simulink library "powerlib_modelsV2"  (Simulink 6.0)
settings: Solver=ode45  SolverMode=SingleTasking  StartTime=0.0  StopTime=10.0  RelTol=1e-3
undefined symbols (not defined in the file or in its folder): A, Ac, B, Bc, C, Cc, Cs, Current, damp, Dc, Dd, DiscIntNeverNeededParam, dref, dwo, exc, F, fb, gate, GH, GHd, GI, GId, GL, GLd, H, HT, hyd, ib, ib2, io, isfinite, j, K, Kd, Kg, L, Lad, Laq, lim, LIM, Ll, Llfd, Llkd, Llkq1, Llkq2, Llr, Lls, LowerFlux, N, N2, Nb, Nb2, nb_arm, p, Par_HarmoA_pu, Par_HarmoB_pu, Par_Timing_Harmo, Par_Timing_Variation, Par_Vps, Pb ... (+58)
libraries: powerlib_extras x14
(part 3 of 11)

== system powerlib_modelsV2/Switch Current Source ==
  IGBT : Subsystem  mask(IGBT model){Ron=0.01, Lon=1e-6, Vf=1, Tf=10e-6, Tt=20e-6, IC=0}
      mask prompts: Ron "Resistance Ron (Ohms) :"; Lon "Inductance Lon (H) :"; Vf "Forward voltage Vf (V) :"; Tf "Current 10% fall time Tf (s) :"; Tt "Current tail time Tt (s):"; IC "Initial current Ic (A) :"
      mask help: Simulink model for the IGBT blockt. In on-state, the IGBT model has an internal resistance (Ron) and an inductance (Lon). Lon cannot be set to zero. In off-state, the IGBT model has an infinite impedance. Discretization of the IGBTblock is available only through the Universal Bridge block.
  detailed_thyristor : Subsystem  mask(Thyristor model){Ron=1e-2, Lon=10e-6, Vf=0.8, IL=0.1, Tq=100e-6, IC=0}
      mask prompts: Ron "Resistance Ron (Ohms) :"; Lon "Inductance Lon (H) :"; Vf "Forward voltage Vf (V) :"; IL "Latching current Il (A) :"; Tq "Turn-off time Tq (s) :"; IC "Initial current Ic (A) :"
      mask help:
      | Simulates a thyristor in parallel with a series Rs-Cs snubber circuit. In on-state thyristor has internal resistance (Ron) and inductance (Lon - required by model, cannot be set to zero). In off-state thyristor impedance is infinite.
      |
      | Input one is Vak and input two is the gate signal .
      | Output one is Iak and output two is the measurement output vector [Iak Vak].
  diode : Subsystem  mask(Diode model){Ron=0.01, Lon=1e-6, Vf=0.8, IC=0}
      mask prompts: Ron "Resistance Ron (Ohms) :"; Lon "Inductance Lon (H) :"; Vf "Forward voltage Vf (V) :"; IC "Initial current Ic (A) :"
      mask help: Simulink model for the Diode block when Lon >0. In on-state, the diode has an internal resistance (Ron) and an inductance (Lon). Lon cannot be set to zero. In off-state, the diode impedance is infinite. Input one is Vak. Output one is Iak and output 2 is the measurement output vector [Iak Vak].
  gto : Subsystem  mask(Gto model){Ron=0.001, Lon=1e-5, Vf=0.8, Tf=200e-6, Tt=200e-6, IC=0}
      mask prompts: Ron "Resistance Ron (Ohms) :"; Lon "Inductance Lon (H) :"; Vf "Forward voltage Vf (V) :"; Tf "Current 10% fall time Tf (s) :"; Tt "Current tail time Tt (s) :"; IC "Initial current Ic (A) :"
      mask help: Simulink model for the GTO block. In on-state, the GTO has an internal resistance (Ron) and an inductance (Lon). Lon cannot be set to zero. In off-state, the GTO impedance is infinite. Input one is Vak and input two is the Gate signal. Output one is Iak and output 2 is the measurement output vector [Iak Vak].
  mosfet : Subsystem  mask(Mosfet model ){Ron=0.001, Lon=0.05, Rd=1e-6, IC=0}
      mask prompts: Ron "MOSFET resistance Ron (Ohms) :"; Lon "MOSFET inductance Lon (H) :"; Rd "Internal diode resistance Rd (Ohms) :"; IC "Initial current Ic (A) :"
      mask help: Simulink model for the MOSFETblock. the model simulate an internal diode in parallel with the MOSFET. In on-state, the MOSFET has an internal resistance (Ron if Ids>0 , Rd if Ids<0) and an inductance (Lon). Lon cannot be set to zero). In off-state, the MOSFET impedance is infinite. Input one is Vds and input two is the Gate signal. Output one is Ids and output 2 is the measurement output vector [Ids Vds].
      mask init:
      | ICmos=abs(IC).*(IC>0);
      | ICdiode=abs(IC).*(IC<0);
  thyristor : Subsystem  AncestorBlock=powerlib_models/Switch Current Source/thyristor_GS  mask(Thyristor s model){Ron=1, Lon=10e-6, Vf=0.8, IC=47e-6}
      mask prompts: Ron "Resistance Ron (Ohms) :"; Lon "Inductance Lon (H) :"; Vf "Forward voltage Vf (V) :"; IC "Initial current Ic (A) :"
      mask help: Simulink model for the Thyristor block when Lon>0. In on-state, the thyristor has an internal resistance (Ron) and an inductance (Lon). Lon cannot be set to zero. In off-state, the thyristor impedance is infinite. Input one is Vak and input two is the gate signal. Output one is Iak and output two is the measurement output vector [Iak Vak].

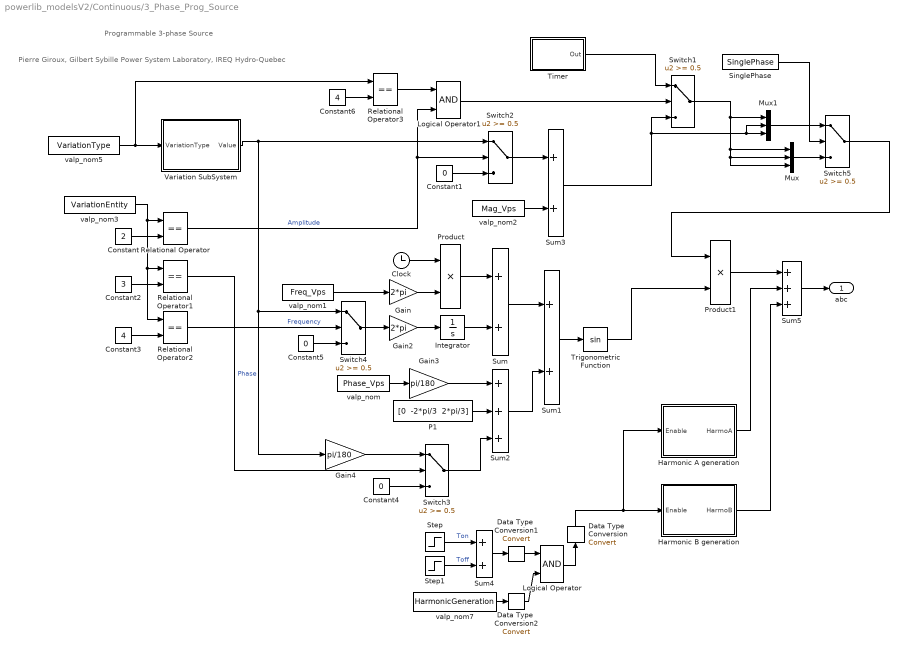
== system powerlib_modelsV2/Continuous/3_Phase_Prog_Source ==
  note: Pierre Giroux, Gilbert Sybille
      | Power System Laboratory, IREQ
      | Hydro-Quebec
  note: Programmable 3-phase Source
  Clock : Clock
  Constant : Constant  Value=2
  Constant1 : Constant  Value=0
  Constant2 : Constant  Value=3
  Constant3 : Constant  Value=4
  Constant4 : Constant  Value=0
  Constant5 : Constant  Value=0
  Constant6 : Constant  Value=4
  Data Type  Conversion : DataTypeConversion  Orientation=up  SaturateOnIntegerOverflow=on  RndMeth=Zero
  Data Type  Conversion1 : DataTypeConversion  SaturateOnIntegerOverflow=on  RndMeth=Zero
  Data Type  Conversion2 : DataTypeConversion  SaturateOnIntegerOverflow=on  RndMeth=Zero
  Gain : Gain  Gain=2*pi  SaturateOnIntegerOverflow=on
  Gain2 : Gain  Gain=2*pi  SaturateOnIntegerOverflow=on
  Gain3 : Gain  Gain=pi/180  SaturateOnIntegerOverflow=on
  Gain4 : Gain  Gain=pi/180  SaturateOnIntegerOverflow=on
  Harmonic A generation : Subsystem  mask(Harmonic generation){Freq_Vps=Freq_Vps, n_Harmo=n_HarmoA, Mag_Harmo=Mag_HarmoA, Phase_Harmo=Phase_HarmoA, Seq_Harmo=Seq_HarmoA, Ts=0}
      mask prompts: Ts "Sample time:"
  Harmonic B generation : Subsystem  mask(Harmonic generation){Freq_Vps=Freq_Vps, n_Harmo=n_HarmoB, Mag_Harmo=Mag_HarmoB, Phase_Harmo=Phase_HarmoB, Seq_Harmo=Seq_HarmoB, Ts=0}
      mask prompts: Ts "Sample time:"
  Integrator : Integrator
  Logical Operator : Logic
  Logical Operator1 : Logic
  Mux : Mux  Inputs=3
  Mux1 : Mux  Inputs=3
  P1 : Constant  Value="[0  -2*pi/3  2*pi/3]"
  Product : Product  SaturateOnIntegerOverflow=on  InputSameDT=on
  Product1 : Product  SaturateOnIntegerOverflow=on  InputSameDT=on
  Relational Operator{,1..3} (4 alike) : RelationalOperator  Operator===  InputSameDT=on
  SinglePhase : Constant  Value=SinglePhase
  Step : Step  Time=Ton_Harmo  SampleTime=0
  Step1 : Step  Time=Toff_Harmo  After=-1  SampleTime=0
  Sum{,1,3..4} (4 alike) : Sum  SaturateOnIntegerOverflow=on  InputSameDT=on
  Sum2 : Sum  Inputs=+++  SaturateOnIntegerOverflow=on  InputSameDT=on
  Sum5 : Sum  Inputs=+++  SaturateOnIntegerOverflow=on  InputSameDT=on
  Switch{1..5} (5 alike) : Switch  Threshold=0.5  InputSameDT=on
  Timer : Subsystem  mask(Timer){t=Xtime, e=Yampli, Ts=0}
      mask prompts: t "Time (s):"; e "Amplitude:"; Ts "Sample time (s)"
      mask help:
      | Generates a signal changing  at specified times.
      |
      | Value of the signal at time zero must  be specified.
      mask init:
      | tt=t;sv=e;
      | tv=[-1,tt(1),reshape(repmat(reshape(tt(2:end),1,length(tt)-1),2,1),1,2*length(tt)-2),tt(end)+1];
      | %sv=(sv(:)'~=0);
      | opv=[sv(1),reshape(repmat(sv(1:end-1),2,1),1,2*length(sv)-2),sv(end),sv(end)];
      mask Display: plot( tv(2:end-1), opv(2:end-1) )
  Trigonometric Function : Trigonometry
  Variation SubSystem : Subsystem  mask(Variation Subsystem){VariationStep=VariationStep, VariationRate=VariationRate, VariationFreq=VariationFreq, VariationMag=VariationMag, Ton_Variation=Ton_Variation, Toff_Variation=Toff_Variation, Ts=0}
      mask prompts: Ts "Sample time:"
  valp_nom : Constant  Value=Phase_Vps
  valp_nom1 : Constant  Value=Freq_Vps
  valp_nom2 : Constant  Value=Mag_Vps
  valp_nom3 : Constant  Value=VariationEntity
  valp_nom5 : Constant  Value=VariationType
  valp_nom7 : Constant  Value=HarmonicGeneration
  abc : Outport  InitialOutput=0
  wires:
  Logical Operator1/1 -> Switch1/2
  Relational Operator3/1 -> Logical Operator1/1
  Switch5/1 -> Product1/1
  Switch1/1 -> Mux1/1, Mux/3, Mux/2, Mux/1
  Mux/1 -> Switch5/3
  SinglePhase/1 -> Switch5/2
  Mux1/1 -> Switch5/1
  Timer/1(Out) -> Switch1/1
  Sum3/1 -> Mux1/2, Mux1/3, Switch1/3
  Constant6/1 -> Relational Operator3/2
  Gain4/1 -> Switch3/1
  Harmonic B generation/1(HarmoB) -> Sum5/3
  Step1/1 -> Sum4/2  "Toff"
  Step/1 -> Sum4/1  "Ton"
  Sum5/1 -> abc/1
  Harmonic A generation/1(HarmoA) -> Sum5/2
  Constant5/1 -> Switch4/3
  Constant3/1 -> Relational Operator2/2
  Constant2/1 -> Relational Operator1/2
  valp_nom3/1 -> Relational Operator1/1, Relational Operator2/1, Relational Operator/1
  Constant/1 -> Relational Operator/2
  Relational Operator2/1 -> Switch4/2  "Frequency"
  Switch4/1 -> Gain2/1
  Variation SubSystem/1(Value) -> Gain4/1, Switch4/1, Switch2/1
  Relational Operator1/1 -> Switch3/2  "Phase"
  Constant4/1 -> Switch3/3
  Switch3/1 -> Sum2/3
  valp_nom5/1 -> Relational Operator3/1, Variation SubSystem/1(VariationType)
  Relational Operator/1 -> Logical Operator1/2, Switch2/2  "Amplitude"
  valp_nom2/1 -> Sum3/2
  Sum2/1 -> Sum1/2
  Constant1/1 -> Switch2/3
  Switch2/1 -> Sum3/1
  Product1/1 -> Sum5/1
  valp_nom1/1 -> Gain/1
  valp_nom/1 -> Gain3/1
  Gain3/1 -> Sum2/1
  Trigonometric Function/1 -> Product1/2
  P1/1 -> Sum2/2
  Integrator/1 -> Sum/2
  Gain2/1 -> Integrator/1
  Sum1/1 -> Trigonometric Function/1
  Sum/1 -> Sum1/1
  Clock/1 -> Product/1
  Gain/1 -> Product/2
  Product/1 -> Sum/1
  Logical Operator/1 -> Data Type  Conversion/1
  Data Type  Conversion/1 -> Harmonic A generation/1(Enable), Harmonic B generation/1(Enable)
  Sum4/1 -> Data Type  Conversion1/1
  Data Type  Conversion1/1 -> Logical Operator/1
  valp_nom7/1 -> Data Type  Conversion2/1
  Data Type  Conversion2/1 -> Logical Operator/2

== system powerlib_modelsV2/Continuous/3_phase_source ==
  Constant : Constant  Value=complex(A*cos(P*pi/180),A*sin(P*pi/180))
  Constant1 : Constant  Value=complex(A*cos((P-120)*pi/180),A*sin((P-120)*pi/180))
  Constant2 : Constant  Value=complex(A*cos((P+120)*pi/180),A*sin((P+120)*pi/180))
  Mux : Mux  Inputs=6
  Sine Wave : Sin  Amplitude=A  Frequency=2*pi*F  Phase=P*pi/180  SampleTime=0
  Sine Wave1 : Sin  Amplitude=A  Frequency=2*pi*F  Phase=(P-120)*pi/180  SampleTime=0
  Sine Wave2 : Sin  Amplitude=A  Frequency=2*pi*F  Phase=(P+120)*pi/180  SampleTime=0
  Out1 : Outport
  wires:
  Constant/1 -> Mux/2
  Sine Wave/1 -> Mux/1
  Sine Wave1/1 -> Mux/3
  Constant1/1 -> Mux/4
  Sine Wave2/1 -> Mux/5
  Constant2/1 -> Mux/6
  Mux/1 -> Out1/1

== system powerlib_modelsV2/Continuous/Dynamic_Load ==
  v : Inport  Port=1  LatchInput=off
  PQ : Inport  Port=2  LatchInput=off
  3-phase PLL1 : Subsystem  mask(3-phase PLL){Par_Init=[Pha_V0  fnom], ParK=[60 1400]}
      mask prompts: Par_Init "Initial inputs:[ Phase(degrees)   Frequency(Hz) ]"; ParK "Regulator gains [ Kp  Ki ]"
      mask help:
      | This Phase Locked Loop (PLL) system can be used  to synchronize on a set of variable frequency, three-phase sinusoidal signals.
      |
      | Input 1: Vector containing the normalized
      |              three-phase signals [Va Vb Vc]
      | Output 1:  Measured frequency (Hz) = w/(2pi)
      | Output 2:  Ramp w.t   varying between  0 and 2*pi,
      | synchronized on zero crossings of the fundamental (positive-sequence) of phase A.
      | Output 3: Vector [sin(wt) cos(wt)]
      mask init:
      | Kp=ParK(1);
      | Ki=ParK(2);
      | Phase_Init=Par_Init(1);
      | Finit=Par_Init(2);
  Break  Alg. Loop : Subsystem  Orientation=left
  Complex to Real-Imag : ComplexToRealImag  Orientation=left
  Demux : Demux  Outputs=2
  Ground : Ground  Orientation=left
  Mux1 : Mux  Orientation=left  Inputs=3
  Positive Sequence  current : Subsystem
  Real-Imag to Complex : RealImagToComplex
  Real-Imag to Complex1 : RealImagToComplex
  Selector : Selector  Orientation=left  Elements=1:2  InputPortWidth=3
  V> pu : Gain  Gain=1/Vbase  SaturateOnIntegerOverflow=on
  Variable Frequency Mean value1 : Subsystem  mask(Variable-Frequency Mean Value){Finit=fnom, Vinit=Mag_V0}
      mask prompts: Finit "Initial frequency (Hz):"; Vinit "Initial input (DC component):"
      mask help:
      | This  block computes the mean value of the input signal (port In) over a running window of one cycle of a specified frequency (port Freq).
      |
      | For the first cycle of simulation (specified by the parameter "Initial frequency"), the ouput is held to the value of the  "Initial input" parameter.
  Variable Frequency Mean value2 : Subsystem  mask(Variable-Frequency Mean Value){Finit=fnom, Vinit=0}
      mask prompts: Finit "Initial frequency (Hz):"; Vinit "Initial input (DC component):"
      mask help:
      | This  block computes the mean value of the input signal (port In) over a running window of one cycle of a specified frequency (port Freq).
      |
      | For the first cycle of simulation (specified by the parameter "Initial frequency"), the ouput is held to the value of the  "Initial input" parameter.
  dq0_to_abc Transformation : Subsystem  Orientation=left  AncestorBlock=powerlib_extras/Measurements/dq0_to_abc Transformation
      mask Type: dq0 to abc Transformation
      mask Description:
      | This block transforms  three quantities  (direct axis, quadature axis and zero-sequence components)  expressed in a two axis reference frame back to phase quantities.
      | 
      | The following transformation is used:
      | 
      | Va = [Vd*sin(wt) +  Vq*cos(wt)  +  Vo ]
      | Vb = [Vd*sin(wt-2pi/3)  + Vq*cos(wt-2pi/3)  + Vo)
      | Vc = [Vd*sin(wt+2pi/3) + Vq*cos(wt+2pi/3)  + Vo)
      | where w=  rotation speed (rad/s) of the rotating frame.
      | 
      | Input 1 contains  the vectorized signal of [Vd Vq  Vo] components
      | Input 2 must contain a  [sin(wt)  cos(wt)] two dimension signal , where w is the rotation speed  of the reference frame.
      | Output is a vectozized signal containing the three  [Va Vb Vc] phase sinusoidal quantities.
      | 
      | Press Help for more information.
      mask Help:
      | This block performs the reverse of the so called Park transformation which is commonly used in three-phase electric machine models. The Park  transformation allows to eliminate time varying inductances by refering the stator and rotor quantities to a fixed or rotating reference frame .
      | In case of a synchrounous machine, the stator quantities are referred to the rotor. Id and Iq represent the two DC currents flowing  in the two equivalent rotor windings ( d winding on the same axis as the field winding, and q winding in quadrature) producing the same flux as the stator Ia, Ib and Ic currents.
      | 
      | See also the abc_to_dq0  block performing the reverse transformation.
  i : Outport  Orientation=left
  m : Outport  Port=2
  wires:
  Selector/1 -> i/1
  v/1 -> V> pu/1
  Break  Alg. Loop/1(Out) -> Complex to Real-Imag/1
  Positive Sequence  current/2(VPQ) -> m/1
  Real-Imag to Complex1/1 -> Positive Sequence  current/2(S_ext)
  Demux/2 -> Real-Imag to Complex1/2
  Demux/1 -> Real-Imag to Complex1/1
  PQ/1 -> Demux/1
  3-phase PLL1/1(Freq) -> Variable Frequency Mean value2/1(Freq), Variable Frequency Mean value1/1(Freq)
  3-phase PLL1/4(Sin_Cos) -> dq0_to_abc Transformation/2(sin_cos)
  3-phase PLL1/2(Vd) -> Variable Frequency Mean value1/2(In)
  Complex to Real-Imag/2 -> Mux1/2
  Complex to Real-Imag/1 -> Mux1/1
  Positive Sequence  current/1(I1(A)) -> Break  Alg. Loop/1(In)
  dq0_to_abc Transformation/1(abc) -> Selector/1
  Variable Frequency Mean value2/1(Mean) -> Real-Imag to Complex/2
  Variable Frequency Mean value1/1(Mean) -> Real-Imag to Complex/1
  Ground/1 -> Mux1/3
  3-phase PLL1/3(Vq) -> Variable Frequency Mean value2/2(In)
  Mux1/1 -> dq0_to_abc Transformation/1(dq0)
  Real-Imag to Complex/1 -> Positive Sequence  current/1(V1(pu))
  V> pu/1 -> 3-phase PLL1/1(Vab_bc (pu))

== system powerlib_modelsV2/Continuous/Excitation_System ==
  vref : Inport  Port=1  LatchInput=off
  vd : Inport  Port=2  LatchInput=off
  vq : Inport  Port=3  LatchInput=off
  vstab : Inport  Port=4  LatchInput=off
  Damping kf.s\ (tf.s +1) : Subsystem  Orientation=left  mask(Transfer Function with Initial Outputs){N=[kf 0], D=[ tf 1], Y0=0, U0=v0(2)}
      mask prompts: N "Numerator:"; D "Denominator:"; Y0 "Initial output:"; U0 "Initial input:"
      mask help: Vector expressions for numerator, and denominator. Coefficients are in descending powers of s.
      mask init:
      | [A,B,C,Dd]=tf2ss(N,D);if (isempty(Y0));[m,n]=size(A);X0=zeros(1,m); end; if (isempty(U0));[m,p]=size(B);U0=zeros(1,p);end;
      |  if isempty(A),  X0=[]; else ,X0=getxo(A,B,C,Dd,U0,Y0,0); end
      mask Help: Specify the initial output for the transfer function.  An optimization routine attempts to determine the appropriate initial states so that the specified initial output is achieved.  For more details, see the m-file getxo.m
      mask Display: dpoly(N,D,'s')
  Exciter 1 \(te.s +ke) : Subsystem  mask(Transfer Function with Initial Outputs){N=1, D=[ te ke], Y0=v0(2), U0=ke*v0(2)}
      mask prompts: N "Numerator:"; D "Denominator:"; Y0 "Initial output:"; U0 "Initial input:"
      mask help: Vector expressions for numerator, and denominator. Coefficients are in descending powers of s.
      mask init:
      | [A,B,C,Dd]=tf2ss(N,D);if (isempty(Y0));[m,n]=size(A);X0=zeros(1,m); end; if (isempty(U0));[m,p]=size(B);U0=zeros(1,p);end;
      |  if isempty(A),  X0=[]; else ,X0=getxo(A,B,C,Dd,U0,Y0,0); end
      mask Help: Specify the initial output for the transfer function.  An optimization routine attempts to determine the appropriate initial states so that the specified initial output is achieved.  For more details, see the m-file getxo.m
      mask Display: dpoly(N,D,'s')
  Lead Lag Compensator tc.s+1\tb.s+1 : Subsystem  mask(Transfer Function with Initial Outputs){N=[tc 1], D=[tb 1], Y0=ke*v0(2)/ka, U0=ke*v0(2)/ka}
      mask prompts: N "Numerator:"; D "Denominator:"; Y0 "Initial output:"; U0 "Initial input:"
      mask help: Vector expressions for numerator, and denominator. Coefficients are in descending powers of s.
      mask init:
      | [A,B,C,Dd]=tf2ss(N,D);if (isempty(Y0));[m,n]=size(A);X0=zeros(1,m); end; if (isempty(U0));[m,p]=size(B);U0=zeros(1,p);end;
      |  if isempty(A),  X0=[]; else ,X0=getxo(A,B,C,Dd,U0,Y0,0); end
      mask Help: Specify the initial output for the transfer function.  An optimization routine attempts to determine the appropriate initial states so that the specified initial output is achieved.  For more details, see the m-file getxo.m
      mask Display: dpoly(N,D,'s')
  Low Pass Filter 1 \ (tr.s+1) (with IC) : Subsystem  mask(Transfer Function with Initial Outputs){N=1, D=[ tr 1], Y0=v0(1), U0=v0(1)}
      mask prompts: N "Numerator:"; D "Denominator:"; Y0 "Initial output:"; U0 "Initial input:"
      mask help: Vector expressions for numerator, and denominator. Coefficients are in descending powers of s.
      mask init:
      | [A,B,C,Dd]=tf2ss(N,D);if (isempty(Y0));[m,n]=size(A);X0=zeros(1,m); end; if (isempty(U0));[m,p]=size(B);U0=zeros(1,p);end;
      |  if isempty(A),  X0=[]; else ,X0=getxo(A,B,C,Dd,U0,Y0,0); end
      mask Help: Specify the initial output for the transfer function.  An optimization routine attempts to determine the appropriate initial states so that the specified initial output is achieved.  For more details, see the m-file getxo.m
      mask Display: dpoly(N,D,'s')
  Main Regulator ka \ (ta.s+1) : Subsystem  mask(Transfer Function with Initial Outputs){N=ka, D=[ ta 1], Y0=ke*v0(2), U0=ke*v0(2)/ka}
      mask prompts: N "Numerator:"; D "Denominator:"; Y0 "Initial output:"; U0 "Initial input:"
      mask help: Vector expressions for numerator, and denominator. Coefficients are in descending powers of s.
      mask init:
      | [A,B,C,Dd]=tf2ss(N,D);if (isempty(Y0));[m,n]=size(A);X0=zeros(1,m); end; if (isempty(U0));[m,p]=size(B);U0=zeros(1,p);end;
      |  if isempty(A),  X0=[]; else ,X0=getxo(A,B,C,Dd,U0,Y0,0); end
      mask Help: Specify the initial output for the transfer function.  An optimization routine attempts to determine the appropriate initial states so that the specified initial output is achieved.  For more details, see the m-file getxo.m
      mask Display: dpoly(N,D,'s')
  Mux : Mux  Inputs=2
  Positive Seqence Voltage : Fcn  Expr=sqrt(u(1)^2 + u(2)^2)
  Sum : Sum  Inputs=++-+-  SaturateOnIntegerOverflow=on  InputSameDT=on
  Vf0 \ ka : Constant  Value=v0(2)/ka
  proportionnal saturation : Subsystem
  Vf : Outport  InitialOutput=0
  wires:
  proportionnal saturation/1(Ef) -> Exciter 1 \(te.s +ke)/1(In1)
  Lead Lag Compensator tc.s+1\tb.s+1/1(Out1) -> Main Regulator ka \ (ta.s+1)/1(In1)
  Sum/1 -> Lead Lag Compensator tc.s+1\tb.s+1/1(In1)
  Positive Seqence Voltage/1 -> Low Pass Filter 1 \ (tr.s+1) (with IC)/1(In1)
  vq/1 -> Mux/2
  vd/1 -> Mux/1
  Mux/1 -> Positive Seqence Voltage/1
  vref/1 -> Sum/1
  vstab/1 -> Sum/4
  Low Pass Filter 1 \ (tr.s+1) (with IC)/1(Out1) -> proportionnal saturation/2(Vtf), Sum/3
  Vf0 \ ka/1 -> Sum/2
  Main Regulator ka \ (ta.s+1)/1(Out1) -> proportionnal saturation/1(Efd)
  Damping kf.s\ (tf.s +1)/1(Out1) -> Sum/5
  Exciter 1 \(te.s +ke)/1(Out1) -> Damping kf.s\ (tf.s +1)/1(In1), Vf/1

== system powerlib_modelsV2/Continuous/GTO-IGBT Bridge ==
  note: GTO:
      |  tail current can be turned off by specifying Tf=0 and Tt=0
  note: Diode Logic :
      | 1) Diodes are blocked when complementary GTOs are switched on
      | 2) When no snubber capacitances are used (Cs=inf), diodes are triggered
      | when complementary GTOs are swithed off
  note: 6
  note: 5
  note: ***********************************************
  note: C
  note: *
      | *
      | ||
      | ||
      | *
      | *
      | *
      | ||
      | ||
      | *
      | *
  note: B
  note: A
  note: Vcc
  note: ***********************************************
  note: 4
  note: 3
  note: *
      | *
      | ||
      | ||
      | *
      | *
      | *
      | ||
      | ||
      | *
      | *
  note: -
  note: +
  note: 2
  note: 1
  note: *
      | *
      | ||
      | ||
      | *
      | *
      | *
      | ||
      | ||
      | *
      | *
  "v " : Inport  Port=1  LatchInput=off
  g : Inport  Port=2  LatchInput=off
  1/Rsw : Gain  Orientation=up  Gain=1./Rsw  SaturateOnIntegerOverflow=on
  2 : Constant  Value=Tf>0 | Tt>0
  Constant1 : Constant  Value=0
  Data Type  Conversion{1,3..5} (4 alike) : DataTypeConversion  SaturateOnIntegerOverflow=on  RndMeth=Zero
  Diode Logic : Subsystem
  GTO Logic : Subsystem
  G_D : Logic  Operator=OR
  Gain : Gain  Orientation=up  Gain=-1  SaturateOnIntegerOverflow=on
  Memory : Memory  InheritSampleTime=on
  Memory1 : Memory  InheritSampleTime=on
  Memory2 : Memory  InheritSampleTime=on
  Product : Product  SaturateOnIntegerOverflow=on  InputSameDT=on
  Relational Operator : RelationalOperator  InputSameDT=on
  "Tail " : Subsystem  TreatAsAtomicUnit=on  mask(Gto tail current){Tf=Tf, Tt=Tt}
      mask prompts: Tf "Current 10% fall time Tf (s) :"; Tt "Current tail time Tt (s) :"
  "Vf " : Subsystem
  iTail : Outport
  Status : Outport  Port=2
  Vf : Outport  Port=3
  wires:
  Memory2/1 -> Vf/1
  GTO Logic/1(status) -> "Vf "/1(status_GTO), Diode Logic/3(G), G_D/2
  "Vf "/1(Vf) -> Memory2/1
  "v "/1 -> Gain/1, GTO Logic/1(Vak), 1/Rsw/1
  "Tail "/1(itail) -> iTail/1
  2/1 -> "Tail "/Enable
  G_D/1 -> Memory/1
  Constant1/1 -> Relational Operator/2
  Memory1/1 -> "Tail "/1(Iak)
  Gain/1 -> Diode Logic/1(Vak)
  Product/1 -> Memory1/1  "IGTO"
  Memory/1 -> Data Type  Conversion1/1
  Data Type  Conversion1/1 -> Status/1
  Data Type  Conversion3/1 -> Product/1
  Relational Operator/1 -> Data Type  Conversion3/1, Diode Logic/2(Ipos)
  g/1 -> Data Type  Conversion4/1
  Data Type  Conversion4/1 -> "Tail "/2(switch), GTO Logic/2(G)
  Diode Logic/1(status) -> Data Type  Conversion5/1
  Data Type  Conversion5/1 -> G_D/1
  1/Rsw/1 -> Relational Operator/1, Product/2

== system powerlib_modelsV2/Continuous/HTG ==
  wref : Inport  Port=1  LatchInput=off
  Pref : Inport  Port=2  LatchInput=off
  we : Inport  Port=3  LatchInput=off
  Pe : Inport  Port=4  LatchInput=off
  dw : Inport  Port=5  LatchInput=off
  Constant1 : Constant  Orientation=left  Value=dref
  PID : Subsystem
      mask Type: PID(2) Controller
      mask Display: disp('PID')
  Sum : Sum  Inputs=+-  SaturateOnIntegerOverflow=on  InputSameDT=on
  Sum1 : Sum  Inputs=+-  SaturateOnIntegerOverflow=on  InputSameDT=on
  Sum5 : Sum  Inputs=-+  SaturateOnIntegerOverflow=on  InputSameDT=on
  Switch : Switch  Orientation=left  Threshold=0.5  InputSameDT=on
  permanent droop : Gain  Orientation=left  Gain=Rp  SaturateOnIntegerOverflow=on
  servo-motor : Subsystem
      mask Display: disp('servo-\nmotor')
  turbine : Subsystem
      mask Display: disp('hydraulic\nturbine')
  Pm : Outport  InitialOutput=0
  gate : Outport  Port=2  InitialOutput=0
  wires:
  Constant1/1 -> Switch/2
  Switch/1 -> permanent droop/1
  Pe/1 -> Sum5/2
  Pref/1 -> Sum5/1
  Sum1/1 -> PID/1(error)
  permanent droop/1 -> Sum1/2
  Sum/1 -> Sum1/1
  PID/1(Output) -> servo-motor/1(regulator's output)
  wref/1 -> Sum/1
  we/1 -> Sum/2
  Sum5/1 -> Switch/3
  servo-motor/1(gate opening) -> turbine/2(gate opening), gate/1, Switch/1
  dw/1 -> turbine/1(dw)
  turbine/1(Pm) -> Pm/1

== system powerlib_modelsV2/Continuous/Impedance Measurement ==
  v : Inport  Port=1  LatchInput=off
  Ground : Ground
  Terminator : Terminator
  i : Outport  InitialOutput=0
  wires:
  Ground/1 -> i/1
  v/1 -> Terminator/1

== system powerlib_modelsV2/Continuous/MBPSS ==
  note: Innocent Kamwa, Robert Grondin
      | IREQ, Hydro-Quebec
  note: Multi-band Power System Stabilizer
  note: (IEEE Type PSS4b)
  note: Note: Speed deviation is derived from the machine positive-sequence terminal voltages and currents.
  note: Low and intermediate speed deviation is based on the internal voltage phasors while
      | the high frequency speed deviation  is based on the electrical power.
  note: (for simplified
      | settings only)
  dw : Inport  Port=1  LatchInput=off
  BF1 : TransferFcn  Numerator=[TL1 KL11]  Denominator=[TL2 1]
  BF7 : TransferFcn  Numerator=[TL7 KL17]  Denominator=[TL8 1]
  Constant : Constant  Value=Detailed
  Gain : Gain  Gain=KL  SaturateOnIntegerOverflow=on
  Gain1 : Gain  Gain=KI  SaturateOnIntegerOverflow=on
  Gain2 : Gain  Gain=KH  SaturateOnIntegerOverflow=on
  Gain3 : Gain  Gain=KL1  SaturateOnIntegerOverflow=on
  Gain4 : Gain  Gain=KL2  SaturateOnIntegerOverflow=on
  Gain5 : Gain  Gain=KI1  SaturateOnIntegerOverflow=on
  Gain6 : Gain  Gain=KI2  SaturateOnIntegerOverflow=on
  Gain7 : Gain  Gain=KH1  SaturateOnIntegerOverflow=on
  Gain8 : Gain  Gain=KH2  SaturateOnIntegerOverflow=on
  Gain9 : Gain  Gain=Kg  SaturateOnIntegerOverflow=on
  HF speed sensor : TransferFcn  Numerator="[80  0 0]"  Denominator=[1 82 161 80]
  HF1 : TransferFcn  Numerator=[TH1 KH11]  Denominator=[TH2 1]
  HF4 : TransferFcn  Numerator=[TH7 KH17]  Denominator=[TH8 1]
  IF1 : TransferFcn  Numerator=[TI1 KI11]  Denominator=[TI2 1]
  IF4 : TransferFcn  Numerator=[TI7 KI17]  Denominator=[TI8 1]
  LF and IF speed sensor : TransferFcn  Numerator=[-1.759e-3 1]  Denominator=[1.2739e-4 1.7823e-2 1]
  "Limiteur BF " : Saturate  UpperLimit=LIM_VL  LowerLimit=-LIM_VL
  Limiteur HF : Saturate  UpperLimit=LIM_VH  LowerLimit=-LIM_VH
  "Limiteur IF " : Saturate  UpperLimit=LIM_VI  LowerLimit=-LIM_VI
  Limiteur VS : Saturate  UpperLimit=LIM_VS  LowerLimit=-LIM_VS
  Sum : Sum  Inputs=+-  SaturateOnIntegerOverflow=on  InputSameDT=on
  Sum1 : Sum  Inputs=+++  SaturateOnIntegerOverflow=on  InputSameDT=on
  Sum2 : Sum  Inputs=+-  SaturateOnIntegerOverflow=on  InputSameDT=on
  Sum3 : Sum  Inputs=+-  SaturateOnIntegerOverflow=on  InputSameDT=on
  Transfer function for detailed model (HF) : Subsystem
  Transfer function for detailed model (IF) : Subsystem
  Transfer function for detailed model (LF) : Subsystem
  VS : Outport  InitialOutput=0
  wires:
  dw/1 -> LF and IF speed sensor/1, HF speed sensor/1
  HF speed sensor/1 -> Gain7/1, Gain8/1
  LF and IF speed sensor/1 -> Gain6/1, Gain5/1, Gain4/1, Gain3/1
  Gain8/1 -> HF4/1
  Gain7/1 -> HF1/1
  Gain6/1 -> IF4/1
  Gain5/1 -> IF1/1
  Gain4/1 -> BF7/1
  Gain3/1 -> BF1/1
  Gain2/1 -> Limiteur HF/1
  Gain1/1 -> "Limiteur IF "/1
  Gain/1 -> "Limiteur BF "/1
  Sum/1 -> Gain/1
  Transfer function for detailed model (LF)/1(LFpos) -> Sum/1
  Transfer function for detailed model (LF)/2(LFneg) -> Sum/2
  BF1/1 -> Transfer function for detailed model (LF)/2("LFpos ")
  BF7/1 -> Transfer function for detailed model (LF)/3("LFneg ")
  Transfer function for detailed model (IF)/1(IFpos) -> Sum2/1
  Transfer function for detailed model (IF)/2(LFneg) -> Sum2/2
  IF1/1 -> Transfer function for detailed model (IF)/2("IFpos ")
  IF4/1 -> Transfer function for detailed model (IF)/3("IFneg ")
  Sum2/1 -> Gain1/1
  HF1/1 -> Transfer function for detailed model (HF)/2("HFpos ")
  HF4/1 -> Transfer function for detailed model (HF)/3("HFneg ")
  Transfer function for detailed model (HF)/1(HFpos) -> Sum3/1
  Transfer function for detailed model (HF)/2(HFneg) -> Sum3/2
  Sum3/1 -> Gain2/1
  "Limiteur BF "/1 -> Sum1/1
  "Limiteur IF "/1 -> Sum1/2
  Limiteur HF/1 -> Sum1/3
  Sum1/1 -> Gain9/1
  Limiteur VS/1 -> VS/1
  Constant/1 -> Transfer function for detailed model (LF)/1(On), Transfer function for detailed model (IF)/1(On), Transfer function for detailed model (HF)/1(On)
  Gain9/1 -> Limiteur VS/1

== system powerlib_modelsV2/Continuous/PM_synchronous_machine ==
  v : Inport  Port=1  LatchInput=off
  Tm : Inport  Port=2  LatchInput=off
  Mux : Mux  Inputs=[3,2,2,3]
  Selector : Selector  Elements=1:2  InputPortWidth=3
  abc2qd : Subsystem
  iq,id : Subsystem
  mec : Subsystem  Orientation=left
  qd2abc : Subsystem
  i : Outport  InitialOutput=0
  m : Outport  Port=2  InitialOutput=0
  wires:
  Selector/1 -> i/1
  qd2abc/1(is) -> Selector/1, Mux/1  "isabc"
  iq,id/1(iq,id) -> qd2abc/2(iq,id), mec/2(iq,id), Mux/2  "iqd"
  v/1 -> abc2qd/1(Vab,Vbc)
  abc2qd/1(s,c) -> qd2abc/1(s,c)
  abc2qd/2(vq,vd) -> iq,id/1(vq,vd), Mux/3  "vqd"
  Mux/1 -> m/1
  mec/1(we) -> iq,id/2(we)
  Tm/1 -> mec/1(Tm)
  mec/3(w,th,Te) -> Mux/4  "w,th,Te"
  mec/2(the) -> abc2qd/2(the)

== system powerlib_modelsV2/Continuous/PSS ==
  note: Power System Stabilizer (PSS)
      | (generic model)
  In : Inport  Port=1  LatchInput=off
  Lead-lag #1 : TransferFcn  Numerator=[T1n 1]  Denominator=[T1d 1]
  Lead-lag #2 : TransferFcn  Numerator=[T2n 1]  Denominator=[T2d 1]
  "Limiter " : Saturate  UpperLimit=VSlimits(2)  LowerLimit=VSlimits(1)
  Overall Gain : Gain  Gain=K  SaturateOnIntegerOverflow=on
  Sensor : Subsystem  AncestorBlock=|  mask(Discrete 1st-Order Filter){FilterType=Lowpass, Tc=Tsensor, Initialize=on, Vac_Init=[0 0 60], Vdc_Init=Vinit, PlotResponse=off, param1=[1 500 1]}
      | powerlib_extras/Control 
      | Blocks/1st-Order 
      | Filter
      mask prompts: FilterType "Filter Type:"; Tc "Time constant (s):"; Initialize "Initialize filter states"; Vac_Init "AC initial input: [ Mag  Phase(degrees)  Freq(Hz) ]"; Vdc_Init "DC Initial input:"; PlotResponse "Plot filter response"; param1 "Frequency range(Hz) : [Start  End  Inc.]"
      mask init:
      | switch FilterType
      | case 1, % Lowpass
      |        X=[0 1 2 3 4];
      |        Y=[-2 -2 -3 -4 -4];
      |        numc=1;
      |        denc=[Tc 1];
      |  case 2,   % Highpass
      |        X=[0 1 2 3 4];
      |        Y=[-4 -4 -3 -2 -2];
      |         numc=[1 0];
      |         denc=[1 1/Tc];
      | end
      | %
      | [Ac,Bc,Cc,Dc]=tf2ss(numc,denc);
      | %
      | %
      | if Initialize==1  % Compute initial conditions on states
      | u1=Vac_Init(1)*exp(j*Vac_Init(2)*pi/180);
      | u2=Vdc_Init*exp(j*90*pi/180);
      | u=u1+u2;
      | u0=imag(u); % input at  t=0;
      | I=eye(size(Ac));
      | sI1=I*j*(2*pi*Vac_Init(3));
      | sI2=I*j*0;
      | x=inv(sI1-Ac)*Bc*u1 + inv(sI2-Ac)*Bc*u2;
      | x0c=imag(x);
      | else
      | x0c=0;
      | end
      | %
      | if PlotResponse==1 % Plot frequency and step response
      | figure(1)
      | sys=ss(Ac,Bc,Cc,Dc);
      | f=param1(1):param1(3):param1(2);
      | w=2*pi*f;
      | [mag phase]=bode(sys,w);
      | subplot(2,1,1)
      | plot(f,squeeze(mag))
      | title('Magnitude')
      | grid
      | subplot(2,1,2)
      | plot(f,squeeze(phase))
      | title('Phase (degrees)')
      | xlabel('Hz')
      | grid
      | figure(2)
      | step(sys)
      | end
      mask StyleString: popup(Lowpass|Highpass),edit,checkbox,edit,edit,checkbox,edit
      mask CallbackString: ||parametres=get_param(gcb,'MaskValues');p3=parametres{3};p6=parametres{6};if strcmp(p3,'on');param4='on';param5='on';else;param4='off';param5='off';end;if strcmp(p6,'on');param7='on';else;param7='off';end;visible={'on','on','on',param4,param5,'on',param7};set_param(gcb,'MaskVisibilities',visible)|||parametres=get_param(gcb,'MaskValues');p3=parametres{3};p6=parametres{6};if strcmp(p3,'on');param4='on';param5='on';else;param4='off';param5='off';end;if strcmp(p6,'on');param7='on';else;param7='off';end;visible={'on','on','on',param4,param5,'on',param7};set_param(gcb,'MaskVisibilities',visible)|
      mask Display: plot(X,Y);
  Wash-out : Subsystem  AncestorBlock=|  mask(Discrete 1st-Order Filter){FilterType=Highpass, Tc=Twashout, Initialize=on, Vac_Init=[0 0 60], Vdc_Init=K*Vinit, PlotResponse=off, param1=[1 500 1]}
      | powerlib_extras/Control 
      | Blocks/1st-Order 
      | Filter
      mask prompts: FilterType "Filter Type:"; Tc "Time constant (s):"; Initialize "Initialize filter states"; Vac_Init "AC initial input: [ Mag  Phase(degrees)  Freq(Hz) ]"; Vdc_Init "DC Initial input:"; PlotResponse "Plot filter response"; param1 "Frequency range(Hz) : [Start  End  Inc.]"
      mask init: same as powerlib_modelsV2/Continuous/PSS/Sensor
      mask StyleString: popup(Lowpass|Highpass),edit,checkbox,edit,edit,checkbox,edit
      mask CallbackString: ||parametres=get_param(gcb,'MaskValues');p3=parametres{3};p6=parametres{6};if strcmp(p3,'on');param4='on';param5='on';else;param4='off';param5='off';end;if strcmp(p6,'on');param7='on';else;param7='off';end;visible={'on','on','on',param4,param5,'on',param7};set_param(gcb,'MaskVisibilities',visible)|||parametres=get_param(gcb,'MaskValues');p3=parametres{3};p6=parametres{6};if strcmp(p3,'on');param4='on';param5='on';else;param4='off';param5='off';end;if strcmp(p6,'on');param7='on';else;param7='off';end;visible={'on','on','on',param4,param5,'on',param7};set_param(gcb,'MaskVisibilities',visible)|
      mask Display: plot(X,Y);
  VS : Outport  InitialOutput=0
  wires:
  "Limiter "/1 -> VS/1
  Lead-lag #2/1 -> "Limiter "/1
  Lead-lag #1/1 -> Lead-lag #2/1
  Wash-out/1(Out) -> Lead-lag #1/1
  Overall Gain/1 -> Wash-out/1(In)
  Sensor/1(Out) -> Overall Gain/1
  In/1 -> Sensor/1(In)

== system powerlib_modelsV2/Continuous/Three-Level Bridge ==
  v : Inport  Port=1  PortDimensions=nb_arm*3  LatchInput=off
  g : Inport  Port=2  PortDimensions=nb_arm*4  LatchInput=off
  2-level GTO-IGBT Bridge  Logic (modified) : Subsystem  AncestorBlock=powerlib_models/Discrete/GTO-IGBT Bridge  mask(GTO & IGBT Bridge Logic(modified)){nb_arm=nb_arm, Tf=0, Tt=0, Cs=Cs, VFs=Par_Vf, Rsw=Ron, Ts=Ts}
      mask prompts: nb_arm "Number of bridge arms (1,2 or 3)"; Tf "Curent 10% fall time Tf (s) :"; Tt "Current tail time Tt (s) :"; Cs "Snubber Capacitance Cs (F):"; VFs "Forward Voltages [ Vf  Vfd ]"; Rsw "Device resistance"; Ts "Time step Ts (s) :"
      mask help:
      | Generates the switch status ( 0 or 1) and the tail currents for a forced-commutated two- level bridge using GTO/Diode or IGBT/Diode pairs.
      | Specify  3 arms (6 switches) for 3 phase bridge, 2 arms for 4 switches, or 1 arm.
      | To turn-off the tail current, specify Tf=0 and Tt=0.
      mask init:
      | Vf=VFs(1);
      | Vfd=VFs(2);
      | nb_switch=nb_arm*2;
      | if nb_arm==1,
      |    Selec_Diode=[2 1];
      |    Block3Elements=[1 2];
      |    VswElements=[1 2];
      | elseif nb_arm==2,
      |    Selec_Diode=[2 1 4 3];
      |    Block3Elements=[1 3 2 4];
      |    VswElements=[1 2 4 5];
      | elseif nb_arm==3,
      |    Selec_Diode=[2 1 4 3 6 5];
      |    Block3Elements=[1 3 5 2 4 6];
      |    VswElements=[1 2 4 5 7 8];
      | end
  Input : Subsystem
  Mux : Mux  Inputs=[nb_arm*2 nb_arm]
  Mux1 : Mux  Inputs=[nb_arm*2 nb_arm]
  Select_Status : Selector  Elements=StatusElements  InputPortWidth=3*nb_arm
  Select_Status1 : Selector  Elements=StatusElements  InputPortWidth=3*nb_arm
  SubSystem : Subsystem
      mask Display: disp('?')
  Sw3 (clamping diode) Logic : Subsystem  mask{nb_arm=nb_arm, VFs=Par_Vf, Ts=Ts}
      mask prompts: nb_arm "Number of bridge arm:"; VFs "Forward Voltages [ Vf  Vfd ]"; Ts "Sample time:"
      mask init:
      | Vf=VFs(1);
      | Vfd=VFs(2);
      | nb_switch=nb_arm*2;
      | if nb_arm==1,
      |    Vsw3Elements=[3];
      |    PulseElements=[1 2 3 4];
      |    g12Elements=[1 2];
      |   Trig12Elements=[1 2];
      | BlockDElements=[1 2];
      | elseif nb_arm==2,
      |    Vsw3Elements=[3 6];
      |    PulseElements=[1 5 2 6 3 7 4 8];
      |    g12Elements=[1 3 2 4];
      |   BlockDElements=[1 3 2 4];
      |   Trig12Elements=[1 3 2 4];
      | elseif nb_arm==3,
      |    Vsw3Elements=[3 6 9];
      |    PulseElements=[1 5 9 2 6 10 3 7 11 4 8 12];
      |    g12Elements=[1 4 2 5 3 6];
      |    BlockDElements=[1 4 2 5 3 6];
      |   Trig12Elements=[1 3 5 2 4 6];
      | end
  x : Outport
  Status : Outport  Port=2
  Vf : Outport  Port=3
  wires:
  2-level GTO-IGBT Bridge  Logic (modified)/4(status_GTO) -> Sw3 (clamping diode) Logic/4(Status_GTO)
  Input/1(Out) -> Sw3 (clamping diode) Logic/2(Pulses)
  g/1 -> Input/1(In)
  Sw3 (clamping diode) Logic/5(Trig12) -> 2-level GTO-IGBT Bridge  Logic (modified)/4(Trig12)
  v/1 -> 2-level GTO-IGBT Bridge  Logic (modified)/1(v), Sw3 (clamping diode) Logic/1(V_Sw123)
  2-level GTO-IGBT Bridge  Logic (modified)/1(status) -> Mux/1
  Mux1/1 -> Select_Status1/1
  Mux/1 -> Select_Status/1
  2-level GTO-IGBT Bridge  Logic (modified)/2(Vf) -> Mux1/1
  Sw3 (clamping diode) Logic/1(Status) -> Mux/2
  Sw3 (clamping diode) Logic/2(Vf) -> Mux1/2
  Sw3 (clamping diode) Logic/3(g12) -> 2-level GTO-IGBT Bridge  Logic (modified)/2(g)
  Sw3 (clamping diode) Logic/4(Block12) -> 2-level GTO-IGBT Bridge  Logic (modified)/3(Block12)
  2-level GTO-IGBT Bridge  Logic (modified)/3(Block3) -> Sw3 (clamping diode) Logic/3(Block3)
  Select_Status/1 -> Status/1
  Select_Status1/1 -> Vf/1, x/1

== system powerlib_modelsV2/Continuous/asynchronous_machine ==
  v : Inport  Port=1  LatchInput=off
  Tm : Inport  Port=2  LatchInput=off
  Gain : Gain  Gain=[ib2*ones(5,1);phib2;phib2;Vb2;Vb2;ib2*ones(5,1);phib2;phib2;Vb2;Vb2;Nb2;Tb2;1]  SaturateOnIntegerOverflow=on
  Mechanical : Subsystem  Orientation=left
      mask Display: disp('Mechanical')
  Mutual fluxes : Subsystem  Orientation=left
  Mux3 : Mux  Inputs=[3,2,2,2,3,2,2,2,3]
  Rotor : Subsystem
      mask Display: disp('Rotor')
  Stator : Subsystem
      mask Display: disp('Stator')
  abc2qd : Subsystem
      mask Display: disp('abc2qd')
  dq2abc : Subsystem
  sin,cos : Subsystem
  i : Outport
  m : Outport  Port=2
  wires:
  sin,cos/2(w-wr) -> Rotor/2(w-wr)
  Mutual fluxes/1(phimq,phimd) -> Rotor/3(phimq,phimd), Stator/1(phimq,phimd)
  sin,cos/1(sin,cos) -> abc2qd/2(sin,cos), dq2abc/1(sin,cos)
  Stator/3(phis,is) -> Mechanical/2(phis,is)
  sin,cos/3(w) -> Stator/3(w)
  abc2qd/2(vqs,vds) -> Stator/2(vqs,vds), Mux3/8
  abc2qd/1(vqr,vdr) -> Rotor/1(vqr,vdr), Mux3/4
  dq2abc/1(irab,isab) -> i/1
  Rotor/2(phiqr,phidr) -> Mutual fluxes/1(phiqr,phidr), Mux3/3
  Rotor/1(iqr,idr) -> Mux3/2, dq2abc/2(iqr,idr)
  v/1 -> abc2qd/1(v)
  Mechanical/2(thr,wr) -> sin,cos/1(thr,wr)
  Stator/1(phiqs,phids) -> Mutual fluxes/2(phiqs,phids), Mux3/7
  Stator/2(iqs,ids) -> dq2abc/3(iqs,ids), Mux3/6
  Mechanical/1(w,Te,thr) -> Mux3/9
  Mux3/1 -> Gain/1
  Gain/1 -> m/1
  dq2abc/3(isabc) -> Mux3/5
  dq2abc/2(irabc) -> Mux3/1
  Tm/1 -> Mechanical/1(Tm)

== system powerlib_modelsV2/Continuous/breaker ==
  v : Inport  Port=1  LatchInput=off
  g : Inport  Port=2  LatchInput=off
  Break Algebraic Loop : Subsystem  mask{Nsw=1, istate=istate}
      mask prompts: Nsw "number of switches"; istate "initial condition"
  Constant : Constant  Value=zeros(Nsw,1)
  S function : S-Function  FunctionName=sfun_psbbreaker  Parameters=istate
  i : Outport  InitialOutput=0
  Status : Outport  Port=2  InitialOutput=0
  wires:
  Constant/1 -> i/1
  v/1 -> S function/1  "Breaker voltage"
  S function/1 -> Break Algebraic Loop/1(In1)  "status"
  g/1 -> S function/2  "gate signal"
  Break Algebraic Loop/1(Out1) -> Status/1

== system powerlib_modelsV2/Continuous/detailed_thyristor (logical) ==
  v : Inport  Port=1  LatchInput=off
  g : Inport  Port=2  LatchInput=off
  0 {1..4} (4 alike) : Constant  Value=0
  1/Rsw : Gain  Orientation=down  Gain=1./Rsw  SaturateOnIntegerOverflow=on
  Break Alg. Loop : Subsystem  mask{Nsw=1}
      mask prompts: Nsw "number of switches"
  Constant : Constant  Value=zeros(Nsw,1)
  Data Type  Conversion{1..4} (4 alike) : DataTypeConversion  SaturateOnIntegerOverflow=on  RndMeth=Zero
  Mux : Mux  Inputs=2
  Saturation : Saturate  UpperLimit=inf  LowerLimit=0
  Sum : Sum  Inputs=|++  SaturateOnIntegerOverflow=on  InputSameDT=on
  Switch : Switch  Threshold=0.5  InputSameDT=on
  b5 : RelationalOperator  Operator=>  InputSameDT=on
  b6 : RelationalOperator  Operator=>  InputSameDT=on
  b7 : RelationalOperator  Operator===  InputSameDT=on
  or2 : Logic  Operator=OR
  or3 : Logic  Inputs=3
  vf : Constant  Value=Vf
  i : Outport  InitialOutput=0
  Status : Outport  Port=2  InitialOutput=0
  m : Outport  Port=3  InitialOutput=0
  Vf : Outport  Port=4  InitialOutput=0
  wires:
  0 2/1 -> b6/2
  or3/1 -> or2/2  "Fire"
  Mux/1 -> m/1  "measurement signals"
  0 3/1 -> b7/2
  or2/1 -> Break Alg. Loop/1(In1)
  Break Alg. Loop/1(Out1) -> Status/1, Switch/2
  0 1/1 -> b5/2
  Constant/1 -> i/1
  v/1 -> Sum/1, b6/1, 1/Rsw/1  "Vak"
  Sum/1 -> Mux/2
  vf/1 -> Vf/1, Sum/2
  Data Type  Conversion4/1 -> or3/2  "Current = 0"
  b5/1 -> Data Type  Conversion1/1
  Data Type  Conversion1/1 -> or2/1  "Current > 0"
  b6/1 -> Data Type  Conversion2/1
  Data Type  Conversion2/1 -> or3/1  "Voltage > 0"
  Data Type  Conversion3/1 -> or3/3  "Gate = 1"
  b7/1 -> Data Type  Conversion4/1
  g/1 -> Data Type  Conversion3/1
  Switch/1 -> Saturation/1
  0 4/1 -> Switch/3
  Saturation/1 -> Mux/1, b7/1, b5/1
  1/Rsw/1 -> Switch/1  "Iak"

== system powerlib_modelsV2/Continuous/diode (logical) ==
  v : Inport  Port=1  LatchInput=off
  0 {1..4} (4 alike) : Constant  Value=0
  Break Alg. Loop : Subsystem  mask{Nsw=1}
      mask prompts: Nsw "number of switches"
  Constant : Constant  Value=zeros(Nsw,1)
  Data Type  Conversion1 : DataTypeConversion  SaturateOnIntegerOverflow=on  RndMeth=Zero
  Data Type  Conversion2 : DataTypeConversion  SaturateOnIntegerOverflow=on  RndMeth=Zero
  Data Type  Conversion3 : DataTypeConversion  SaturateOnIntegerOverflow=on  RndMeth=Zero
  Gain : Gain  Gain=1./Rsw  SaturateOnIntegerOverflow=on
  Mux : Mux  Inputs=2
  Saturation : Saturate  UpperLimit=inf  LowerLimit=0
  Sum : Sum  Inputs=|++  SaturateOnIntegerOverflow=on  InputSameDT=on
  Switch : Switch  Threshold=0.5  InputSameDT=on
  b5 : RelationalOperator  Operator=>  InputSameDT=on
  b6 : RelationalOperator  Operator=>  InputSameDT=on
  b7 : RelationalOperator  Operator===  InputSameDT=on
  or2 : Logic  Operator=OR
  or3 : Logic
  vf : Constant  Value=Vf
  i : Outport  InitialOutput=0
  status : Outport  Port=2  InitialOutput=0
  m : Outport  Port=3  InitialOutput=0
  Vf : Outport  Port=4  InitialOutput=0
  wires:
  0 3/1 -> b7/2
  0 2/1 -> b6/2
  v/1 -> b6/1, Gain/1, Sum/1  "Diode voltage"
  Mux/1 -> m/1  "measurement signals"
  b6/1 -> Data Type  Conversion2/1  "Voltage > 0"
  or3/1 -> or2/2
  or2/1 -> Break Alg. Loop/1(In1)
  Break Alg. Loop/1(Out1) -> status/1, Switch/2  "status"
  0 4/1 -> b5/2
  b5/1 -> Data Type  Conversion1/1  "Current > 0"
  Constant/1 -> i/1
  Sum/1 -> Mux/2  "V = Vak + Vf"
  vf/1 -> Sum/2, Vf/1
  b7/1 -> Data Type  Conversion3/1  "Current = 0"
  Data Type  Conversion1/1 -> or2/1
  Data Type  Conversion2/1 -> or3/1
  Data Type  Conversion3/1 -> or3/2
  Switch/1 -> Saturation/1
  0 1/1 -> Switch/3
  Saturation/1 -> Mux/1, b7/1, b5/1  "Diode current"
  Gain/1 -> Switch/1  "Diode current"

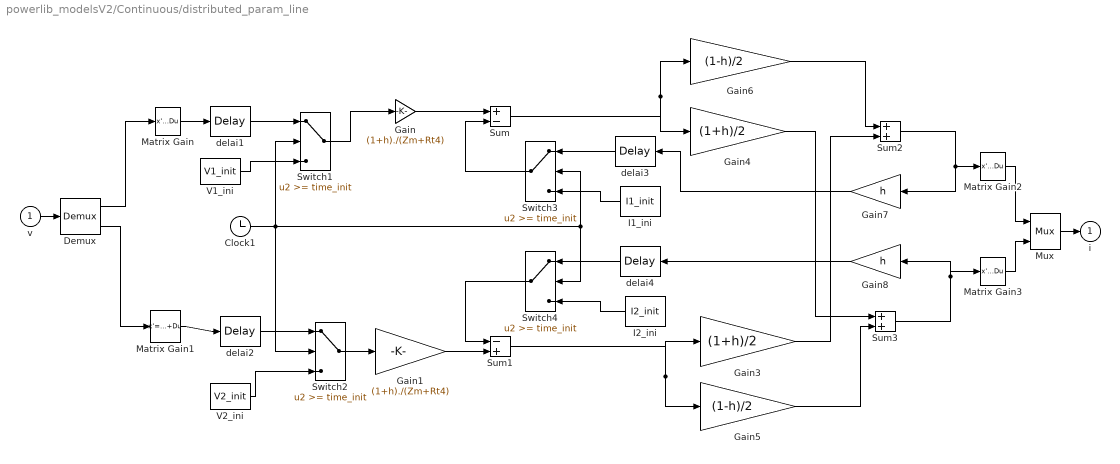
== system powerlib_modelsV2/Continuous/distributed_param_line ==
  v : Inport  Port=1  LatchInput=off
  Clock1 : Clock
      settings: Decimation=10
  Demux : Demux  Outputs=[nphase,nphase]
  Gain : Gain  Gain=(1+h)./(Zm+Rt4)  SaturateOnIntegerOverflow=on
  Gain1 : Gain  Gain=(1+h)./(Zm+Rt4)  SaturateOnIntegerOverflow=on
  Gain3 : Gain  Gain=(1+h)/2  SaturateOnIntegerOverflow=on
  Gain4 : Gain  Gain=(1+h)/2  SaturateOnIntegerOverflow=on
  Gain5 : Gain  Gain=(1-h)/2  SaturateOnIntegerOverflow=on
  Gain6 : Gain  Gain=(1-h)/2  SaturateOnIntegerOverflow=on
  Gain7 : Gain  Orientation=left  Gain=h  SaturateOnIntegerOverflow=on
  Gain8 : Gain  Orientation=left  Gain=h  SaturateOnIntegerOverflow=on
  I1_ini : FromWorkspace  Orientation=left  VariableName=I1_init  SampleTime=0
  I2_ini : FromWorkspace  Orientation=left  VariableName=I2_init  SampleTime=0
  Matrix Gain : StateSpace  A=[]  B=[]  C=[]  D=K  mask(Matrix Gain){@1=Ti'}
      mask prompts: @1 "Gain matrix:"
      mask help: Matrix Gain.
      mask init:
      | K = @1;
      mask Help: Multiplies input vector by entered matrix to produce output vector (y=Au).
      mask Display: disp('K')
  Matrix Gain1 : StateSpace  A=[]  B=[]  C=[]  D=K  mask(Matrix Gain){@1=Ti'}
      mask prompts: @1 "Gain matrix:"
      mask help: Matrix Gain.
      mask init:
      | K = @1;
      mask Help: Multiplies input vector by entered matrix to produce output vector (y=Au).
      mask Display: disp('K')
  Matrix Gain2 : StateSpace  A=[]  B=[]  C=[]  D=K  mask(Matrix Gain){@1=Ti}
      mask prompts: @1 "Gain matrix:"
      mask help: Matrix Gain.
      mask init:
      | K = @1;
      mask Help: Multiplies input vector by entered matrix to produce output vector (y=Au).
      mask Display: disp('K')
  Matrix Gain3 : StateSpace  A=[]  B=[]  C=[]  D=K  mask(Matrix Gain){@1=Ti}
      mask prompts: @1 "Gain matrix:"
      mask help: Matrix Gain.
      mask init:
      | K = @1;
      mask Help: Multiplies input vector by entered matrix to produce output vector (y=Au).
      mask Display: disp('K')
  Mux : Mux  Inputs=[nphase,nphase]
  Sum : Sum  Inputs=+-  SaturateOnIntegerOverflow=on  InputSameDT=on
  Sum1 : Sum  Inputs=-+  SaturateOnIntegerOverflow=on  InputSameDT=on
  Sum2 : Sum  SaturateOnIntegerOverflow=on  InputSameDT=on
  Sum3 : Sum  SaturateOnIntegerOverflow=on  InputSameDT=on
  Switch1 : Switch  Threshold=time_init  InputSameDT=on
  Switch2 : Switch  Threshold=time_init  InputSameDT=on
  Switch3 : Switch  Orientation=left  Threshold=time_init  InputSameDT=on
  Switch4 : Switch  Orientation=left  Threshold=time_init  InputSameDT=on
  V1_ini : FromWorkspace  VariableName=V1_init  SampleTime=0
  V2_ini : FromWorkspace  VariableName=V2_init  SampleTime=0
  delai1 : TransportDelay  DelayTime=to
  delai2 : TransportDelay  DelayTime=to
  delai3 : TransportDelay  Orientation=left  DelayTime=to
  delai4 : TransportDelay  Orientation=left  DelayTime=to
  i : Outport  InitialOutput=0
  wires:
  Matrix Gain2/1 -> Mux/1
  Matrix Gain3/1 -> Mux/2
  Demux/2 -> Matrix Gain1/1
  Matrix Gain1/1 -> delai2/1
  Demux/1 -> Matrix Gain/1
  Matrix Gain/1 -> delai1/1
  Gain4/1 -> Sum3/1
  Gain3/1 -> Sum2/2
  Gain6/1 -> Sum2/1
  Gain5/1 -> Sum3/2
  Gain/1 -> Sum/1
  Gain1/1 -> Sum1/2
  v/1 -> Demux/1
  Mux/1 -> i/1
  Sum3/1 -> Gain8/1, Matrix Gain3/1
  Gain7/1 -> delai3/1
  Sum2/1 -> Gain7/1, Matrix Gain2/1
  Gain8/1 -> delai4/1
  delai1/1 -> Switch1/1
  V1_ini/1 -> Switch1/3
  Switch2/1 -> Gain1/1
  Switch1/1 -> Gain/1
  delai2/1 -> Switch2/1
  V2_ini/1 -> Switch2/3
  Sum/1 -> Gain4/1, Gain6/1
  Sum1/1 -> Gain3/1, Gain5/1
  delai3/1 -> Switch3/1
  Switch3/1 -> Sum/2
  Switch4/1 -> Sum1/1
  delai4/1 -> Switch4/1
  Clock1/1 -> Switch4/2, Switch3/2, Switch2/2, Switch1/2
  I1_ini/1 -> Switch3/3
  I2_ini/1 -> Switch4/3

== system powerlib_modelsV2/Continuous/hysteresis_transformer ==
  v : Inport  Port=1  LatchInput=off
  Hysteresis ( always SI ) : Subsystem
  fluxinit : Integrator  InitialCondition=fluxinit
  i : Outport  InitialOutput=0
  f : Outport  Port=2  InitialOutput=0
  wires:
  Hysteresis ( always SI )/1(Out1) -> i/1
  v/1 -> fluxinit/1
  fluxinit/1 -> Hysteresis ( always SI )/1(In1), f/1  "flux displayed by Multimeter block"

== system powerlib_modelsV2/Continuous/ideal_switch ==
  v : Inport  Port=1  LatchInput=off
  g : Inport  Port=2  LatchInput=off
  0 1 : Constant  Value=0
  1/Rsw : Gain  Gain=1./Rsw  SaturateOnIntegerOverflow=on
  Constant : Constant  Value=zeros(Nsw,1)
  Data Type Conversion : DataTypeConversion  SaturateOnIntegerOverflow=on  RndMeth=Zero
  Mux : Mux  Inputs=2
  Switch : Switch  Threshold=0.5  InputSameDT=on
  i : Outport  InitialOutput=0
  Status : Outport  Port=2  InitialOutput=0
  m : Outport  Port=3  InitialOutput=0
  wires:
  g/1 -> Switch/2, Data Type Conversion/1
  Mux/1 -> m/1  "measurement signals"
  v/1 -> Mux/2, 1/Rsw/1  "Vak"
  Constant/1 -> i/1
  1/Rsw/1 -> Switch/1  "Iak"
  Switch/1 -> Mux/1
  0 1/1 -> Switch/3
  Data Type Conversion/1 -> Status/1

== system powerlib_modelsV2/Continuous/saturable_transformer ==
  v : Inport  Port=1  LatchInput=off
  Integrator : Integrator  InitialCondition=fluxinit
  Look-Up Table : Lookup  DialogController=Simulink.DDGSource  InputValues=phisat  OutputValues=isat  SaturateOnIntegerOverflow=on
  i : Outport  InitialOutput=0
  f : Outport  Port=2  InitialOutput=0
  wires:
  Look-Up Table/1 -> i/1
  v/1 -> Integrator/1
  Integrator/1 -> Look-Up Table/1, f/1
